simulink library "PIDContrallerLib"  (R2022b)
settings: Solver=VariableStepAuto  StartTime=0.0  StopTime=10.0  RelTol=1e-3
undefined symbols (not defined in the file or in its folder): K_D, K_I, K_P, Ts
settings Model: Creator=yasso  LastModifiedBy=yasso

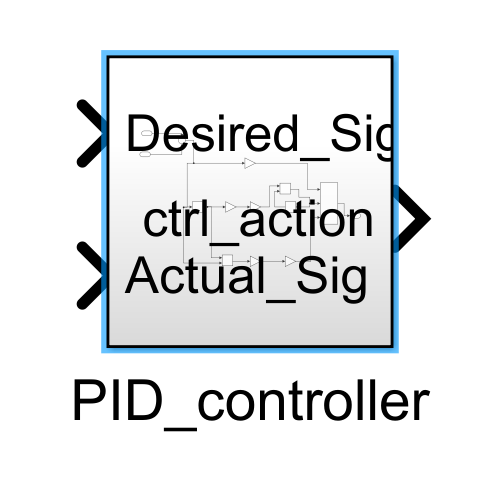
[thumbnail: Simulink's stored preview of the top-level diagram]
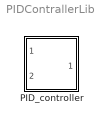
== system PIDContrallerLib ==
  PID_controller : Subsystem

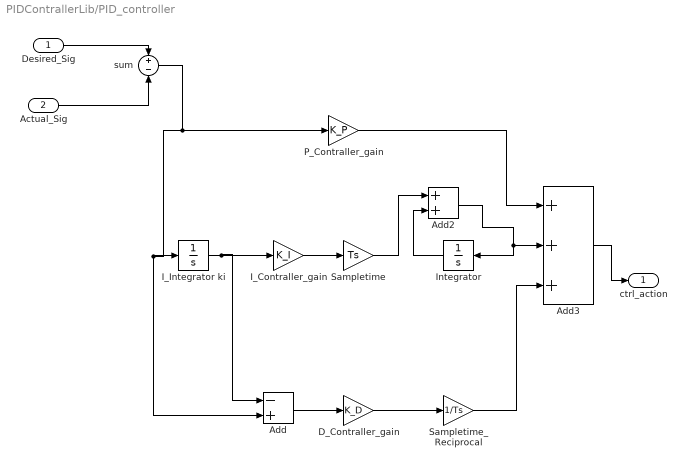
== system PIDContrallerLib/PID_controller ==
  Desired_Sig : Inport
  Actual_Sig : Inport  Port=2
  Add : Sum  Inputs=-+
  Add2 : Sum
  Add3 : Sum  Inputs=+++
  D_Contraller_gain : Gain  Gain=K_D
  I_Contraller_gain : Gain  Gain=K_I
  I_Integrator ki : Integrator
  Integrator : Integrator
  P_Contraller_gain : Gain  Gain=K_P
  Sampletime : Gain  Gain=Ts
  Sampletime_Reciprocal : Gain  Gain=1/Ts
  sum : Sum  Inputs=+-
  ctrl_action : Outport
  wires:
  Desired_Sig/1 -> sum/1
  Actual_Sig/1 -> sum/2
  sum/1 -> I_Integrator ki/1, Add/2, P_Contraller_gain/1
  P_Contraller_gain/1 -> Add3/1
  I_Integrator ki/1 -> Add/1, I_Contraller_gain/1
  I_Contraller_gain/1 -> Sampletime/1
  Sampletime/1 -> Add2/1
  Add2/1 -> Integrator/1, Add3/2
  Integrator/1 -> Add2/2
  Add/1 -> D_Contraller_gain/1
  D_Contraller_gain/1 -> Sampletime_Reciprocal/1
  Sampletime_Reciprocal/1 -> Add3/3
  Add3/1 -> ctrl_action/1
